simulink model "Model2_sat"  (R2018b)
settings: Solver=VariableStepAuto  StartTime=0.0  StopTime=T  RelTol=1e-3
values from neighbouring files (symbols this model uses):
  D_ = [0 0]    [7_8.m]    (also in CEEProject.m; CEEproject.m; Ines.m; MCsynthesis.m)
  L = lqe(A, G, C, Qe, Re)    [7_8.m]    (also in CEEProject.m; CEEproject.m; Ines.m; MCsynthesis.m)
  V = A - B*K - L*C    [7_8.m]    (also in CEEProject.m; CEEproject.m; Ines.m; MCsynthesis.m)
  x0 = [pi,0,0.1,0,0]'    [7_8.m]    (also in CEEProject.m = [pi/4,0,0.18,0,0]'; CEEproject.m = [0.1,0,0,0,0]'; Ines.m = [pi,0,0.4,0,0]'; MCsynthesis.m = [pi/2,0,0.18,0,0]')
undefined symbols (not defined in the file or in its folder): A, B, C, D, K
settings Model: Creator=miguelsilva  LastModifiedBy=miguelsilva

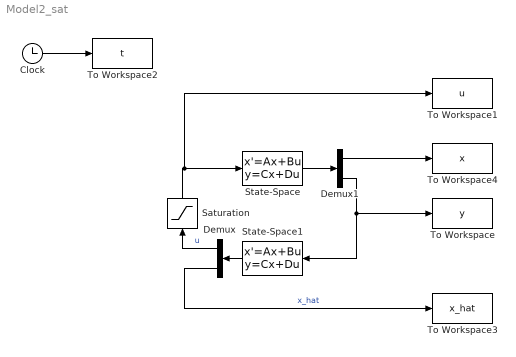
== system Model2_sat ==
  Clock : Clock
  Demux : Demux  Outputs=2
  Demux1 : Demux  Outputs=2
  Saturation : Saturate  UpperLimit=5  LowerLimit=-5
  State-Space : StateSpace  A=A  B=B  C=[eye(5);C]  D=[zeros(5,1);D]  InitialCondition=x0  ContinuousStateAttributes={'x1','x2','x3','x4','x5'}
  State-Space1 : StateSpace  A=V  B=L  C=[-K; eye(5)]  D=[D_;zeros(5,2)]  InitialCondition=0  ContinuousStateAttributes={'y1','y2','y3','y4','y5'}
  To Workspace : ToWorkspace  VariableName=y  SampleTime=-1
  To Workspace1 : ToWorkspace  VariableName=u  SampleTime=-1
  To Workspace2 : ToWorkspace  VariableName=t  SampleTime=-1
  To Workspace3 : ToWorkspace  VariableName=x_hat  SampleTime=-1
  To Workspace4 : ToWorkspace  VariableName=x  SampleTime=-1
  wires:
  Clock/1 -> To Workspace2/1
  State-Space1/1 -> Demux/1
  Demux/1 -> Saturation/1  "u"
  Demux/2 -> To Workspace3/1  "x_hat"
  State-Space/1 -> Demux1/1
  Demux1/1 -> To Workspace4/1
  Saturation/1 -> State-Space/1, To Workspace1/1
  Demux1/2 -> To Workspace/1, State-Space1/1
